simulink model "HyL_SV_test"  (R2013a)
settings: Solver=ode45  StartTime=0.0  StopTime=3  FixedStep=1e-3  MinStep=1e-3  RelTol=1e-3
model workspace (MATLAB code in the model file):
  | % Data obtained from:
  | % ------------------------------------------------------------
  | % HyQ-Robot: Standard Definition for Joint Angles
  | % and Kinematic Parameters of the Legs and Torso
  | %
  | % Project: HyQ-Robot V1.0 with Leg V2.0
  | % Genoa, 9th July 2010
  | %-------------------------------------------------------------
  | % This Matlab file was made by:
  | % Job Ledezma
  | % Genova, Feb 2016
  | %-------------------------------------------------------------
  | 
  | 
  | % ________________________________________
  | %
  | %                HYL DESCRIPTION PARAMETERS
  | %________________________________________
  | 
  | % ---- Leg data ------
  | 
  | m1 = 1.772;              % Kg - Upper leg mass
  | m2 = 0.808;              % Kg - Lower leg mass
  | M = 3.982;                % Kg - Base mass
  | P_01 = 0.08;             % m - distance P0-P1
  | P_12 = 0.350;           % m - distance P1-P2
  | P_23 = 0.330;           % m - distance P2-P3
  | FR = 0.02;                 % m - foot radius
  | P1m1 = 0.164;           % m - distance P1-Pm1
  | P2m2 = 0.122;           % m - distance P2-Pm2
  | I1zz = 0.0713;           % kg·m2 - Inertia upper leg
  | I2zz = 0.0218;           % kg·m2 - Inertia lower leg
  | em1 = deg2rad(7.9);  % rad
  | em2 = deg2rad(0);     % rad
  | g  = 9.810;                 % m/s2 - gravity
  | 
  | % ----- Lever Arm Parameters -----
  | 
  | % Hip joint
  | a1   = 0.3219;             % m
  | b1   = 0.045;               % m
  | e11 = deg2rad(6.24); % rad
  | e12 = deg2rad(0);      % rad
  | 
  | % Knee joint
  | a2 = 0.3218;               % m
  | b2 = 0.045;                 % m
  | e21 = deg2rad(8.04);  % rad
  | e22 = deg2rad(6);       % rad
  | 
  | % ----- Limit Angles --------
  | 
  | % Initial conditions
  | q0_0 = 1;                           % m - height of the floating base
  | q1_0 = deg2rad(45);         % rad - HFE angle
  | q2_0 = deg2rad(-90);        % rad - KFE angle
  | 
  | % Max angle limits
  | q1Max = deg2rad(70);       % rad
  | q2Max = deg2rad(-20);      % rad
  | 
  | % Min angle limits
  | q1Min = deg2rad(-50);        % rad
  | q2Min = deg2rad(-140);      % rad
  | q0Min = P_01+P_12*cos(q1Min)+P_23*cos(q1Min+q2Min)+FR;     % m
  | 
  | % ________________________________________________________
  | %
  | %                                        HYDRAULIC PARAMETERS
  | % ________________________________________________________
  | 
  | % ------ Power unit --------
  | 
  | ps  = 160e5;                            % Pa - Supply pressure
  | pt  = 10e5;                              % Pa - Tank pressure
  | dpt = ps - pt;                           % Pa - Delta pressure
  | beta = 1.4e9;                          % Pa- Effective bulk modulus
  | 
  | % Initial condition for Pressure integrators
  | pAo = ps/2;
  | pBo = ps/2;
  | 
  | %----- Cylinder - HOERBIGER LB6 16 10 0080 4M ----------
  | 
  | Dp = 0.016;                             % m - Piston diameter
  | Dr = 0.010;                              % m - Rod diameter
  | L  = 0.080;                               % m- Stroke
  | Aa = pi*(Dp^2)/4;                   % m^2 - Area A of the piston
  | Ab = pi*(Dp^2-Dr^2)/4;         % m^2 - Area B of the piston
  | r  = Aa/Ab;                              % Relation between areas
  | fv = 700;                                 %  Ns/m - Viscous friction
  | % leak = 1.7*10^-13;            % m3/(s.Pa) - Cylinder leakage
  | Mp = ((pi*Dr^2/4)*L + Aa*0.15)*7860;    % Kg - Piston mass (approximated)
  | 
  | %-----  Valve Parameters - MOOG E024 - 177LA ----------
  | 
  | Un   = 10;                              % V - Nominal tension
  | Qn   = 5 / 60e3;                    % m^3/s - Nominal flow rate
  | dptn = 70e5;                         % Pa - Valve pressure drop
  | Qlk   = 0.28 / 60e3;               % m^3/s - Leakage flow
  | Plk    = 210e5;                       % Pa - Nominal supply pressure for leakage test
  | wn    = 2*32*pi;                    % rad/s - Valve's natural frequency
  | E       = 0.9;                           % Valve's damping coefficient
  | Kv     = Qn/sqrt(dptn);          % m^3/(s*sqrt(Pa)) - Total flow coefficient
  | Kva    = Kv*sqrt(2);               % m^3/(s*sqrt(Pa)) - Partial flow coefficient A
  | Kvb    = Kv*sqrt(2);               % m^3/(s*sqrt(Pa)) - Partial flow coefficient B
  | Kvlk   = Qlk/sqrt(2*Plk);         % m^3/(s*sqrt(Pa)) - Total leakage flow coefficient
  | KvlkA  = Kvlk;                         % m^3/(s*sqrt(Pa)) -  Partial leakage flow coefficient A
  | KvlkB  = Kvlk;                         % m^3/(s*sqrt(Pa)) - Partial leakage flow coefficient B
  | 
  | %------------   Manifold  -----------
  | % Review this part with the manifold's CAD design
  | 
  | v1a = (pi*(0.0035^2)/4)*0.07255;
  | v2a = (pi*(0.006^2)/4)*(0.090-0.012);
  | v1b = (pi*(0.0035^2)/4)*0.04491;
  | v2b = (pi*(0.006^2)/4)*(0.019+0.009);
  | v3b = (pi*(0.006^2)/4)*(0.007+0.009);
  | V0A = v1a + v2a;                                            % Dead volume coupled to chamber A
  | V0B = v1b + v2b + v3b;                                  % Dead volume coupled to chamber B
  | 
  | %-------  Load cell - BURSTER 8417-6005 ----------
  | 
  | xs = 6e-6;                             % m - Maximum deflection @ full scale
  | Fs = 5000;                             % N - Maximum force
  | Ks = Fs / xs ;                         % N·m - Load cell stiffness
  | 
  | %------ Accumulator - FOX-ITALY HST 0,04 ----------
  | 
  | acc = 0;
  | 
  | n = 1.4;                                % Polytropic constant
  | V0 = 0.04e-3;                       % m3 - Initial volume
  | P0 = 120e5 + 1e5;               % Pa - Precharge pressure
  | Cex = 0;                                % m3/Pa - External flowrate coefficient between chambers (in case of damping requirement)
undefined symbols (not defined in the file): Fpt, gcontact, gcPosVel, HyL_Job
libraries: simulink x4
settings Model: Creator=Toshiba  LastModifiedBy=Toshiba
settings SolverCC: ZeroCrossControl=EnableAll  ZeroCrossAlgorithm=Adaptive

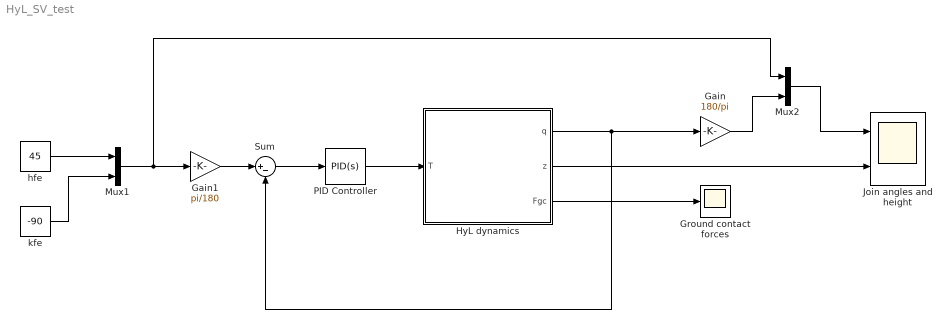
== system HyL_SV_test ==
  Gain : Gain  Gain=180/pi
  Gain1 : Gain  Gain=pi/180
  Ground contact forces : Scope
      settings: SaveName=ScopeData3
  HyL dynamics : Subsystem
  Join angles and height : Scope  NumInputPorts=2
      settings: YMin=-150~-1.14399e-05  YMax=75~-1.03503e-05
  Mux1 : Mux  Inputs=2
  Mux2 : Mux  Inputs=2
  PID Controller : simulink/Continuous/PID Controller  Controller=PID  TimeDomain=Continuous-time  SampleTime=1  IntegratorMethod=Forward Euler  FilterMethod=Forward Euler  Form=Parallel  P=200  I=0  D=6  N=100  InitialConditionSource=internal  InitialConditionForIntegrator=0  InitialConditionForFilter=0  ExternalReset=none  LimitOutput=off  UpperSaturationLimit=inf  LowerSaturationLimit=-inf  LinearizeAsGain=on  AntiWindupMode=none  Kb=1  TrackingMode=off  Kt=1  PParamMin=[]  PParamMax=[]  IParamMin=[]  IParamMax=[]  DParamMin=[]  DParamMax=[]  NParamMin=[]  NParamMax=[]  KbParamMin=[]  KbParamMax=[]  KtParamMin=[]  KtParamMax=[]  POutMin=[]  POutMax=[]  IOutMin=[]  IOutMax=[]  DOutMin=[]  DOutMax=[]  NOutMin=[]  NOutMax=[]  KbOutMin=[]  KbOutMax=[]  KtOutMin=[]  KtOutMax=[]  IntegratorOutMin=[]  IntegratorOutMax=[]  FilterOutMin=[]  FilterOutMax=[]  SumOutMin=[]  SumOutMax=[]  SumI1OutMin=[]  SumI1OutMax=[]  SumI2OutMin=[]  SumI2OutMax=[]  SumI3OutMin=[]  SumI3OutMax=[]  SumDOutMin=[]  SumDOutMax=[]  SaturationOutMin=[]  SaturationOutMax=[]  IntegratorContinuousStateAttributes=''  IntegratorStateMustResolveToSignalObject=off  IntegratorRTWStateStorageClass=Auto  FilterContinuousStateAttributes=''  FilterStateMustResolveToSignalObject=off  FilterRTWStateStorageClass=Auto
  Sum : Sum  Inputs=|+-
  hfe : Constant  Value=45
  kfe : Constant  Value=-90
  wires:
  HyL dynamics/1(q) -> Gain/1, Sum/2
  HyL dynamics/2(z) -> Join angles and height/2
  Mux1/1 -> Mux2/1, Gain1/1
  kfe/1 -> Mux1/2
  hfe/1 -> Mux1/1
  Sum/1 -> PID Controller/1
  Gain1/1 -> Sum/1
  Gain/1 -> Mux2/2
  Mux2/1 -> Join angles and height/1
  HyL dynamics/3(Fgc) -> Ground contact forces/1
  PID Controller/1 -> HyL dynamics/1(T)

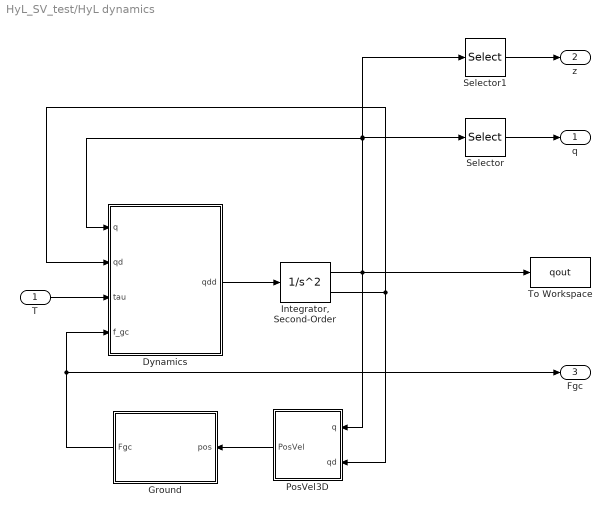
== system HyL_SV_test/HyL dynamics ==
  T : Inport
  Dynamics : Subsystem
  Ground : Subsystem
  "Integrator, Second-Order" : SecondOrderIntegrator  ICX=[q0_0;q1_0;q2_0]  LimitX=on  UpperLimitX=[inf; q1Max; q2Max]  LowerLimitX=[q0Min; q1Min; q2Min]
  PosVel3D : Subsystem
  Selector : Selector  InputPortWidth=3  IndexOptions=Index vector (dialog)  Indices=[2 3]  OutputSizes=1
  Selector1 : Selector  InputPortWidth=3  IndexOptions=Index vector (dialog)  Indices=1  OutputSizes=1
  To Workspace : ToWorkspace  VariableName=qout  SampleTime=-1  SaveFormat=Timeseries
  q : Outport
  z : Outport  Port=2
  Fgc : Outport  Port=3
  wires:
  Dynamics/1(qdd) -> "Integrator, Second-Order"/1
  "Integrator, Second-Order"/1 -> Selector1/1, Selector/1, Dynamics/1(q), To Workspace/1, PosVel3D/1(q)
  "Integrator, Second-Order"/2 -> PosVel3D/2(qd), Dynamics/2(qd)
  Selector/1 -> q/1
  T/1 -> Dynamics/3(tau)
  Selector1/1 -> z/1
  PosVel3D/1(PosVel) -> Ground/1(pos)
  Ground/1(Fgc) -> Fgc/1, Dynamics/4(f_gc)

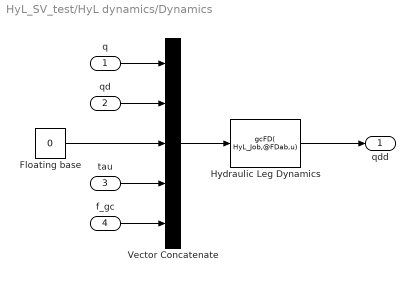
== system HyL_SV_test/HyL dynamics/Dynamics ==
  q : Inport
  qd : Inport  Port=2
  tau : Inport  Port=3
  f_gc : Inport  Port=4
  Floating base : Constant  Value=0
  Hydraulic Leg Dynamics : MATLABFcn  MATLABFcn=gcFD( HyL_Job,@FDab,u)  OutputDimensions=[3 1]  OutputSignalType=real  Output1D=off
  Vector Concatenate : Concatenate  NumInputs=5
  qdd : Outport
  wires:
  Hydraulic Leg Dynamics/1 -> qdd/1
  Vector Concatenate/1 -> Hydraulic Leg Dynamics/1
  qd/1 -> Vector Concatenate/2
  q/1 -> Vector Concatenate/1
  f_gc/1 -> Vector Concatenate/5
  tau/1 -> Vector Concatenate/4
  Floating base/1 -> Vector Concatenate/3

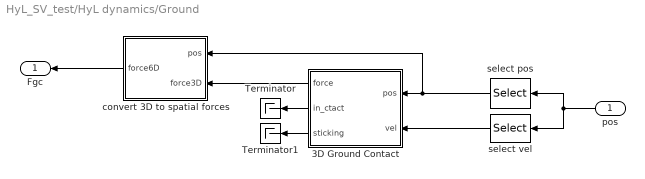
== system HyL_SV_test/HyL dynamics/Ground ==
  pos : Inport
  3D Ground Contact : Subsystem  mask(3D Nonlinear Ground Contact with Friction){K=1e6, D=2000, mu=0.1, np=1}
      mask prompts: K "Stiffness (K)"; D "Damping (D)"; mu "Coefficient of Friction (mu)"; np "Number of Contact Points"
      mask help:
      | Given two 3xnp arrays containing contact-point positions and
      | velocities, calculate the 3xnp array of ground-reaction forces
      | acting on those points. Also calculate 1xnp boolean vectors
      | in_ctact (true if normal force >0) and sticking (true if inside
      | or on boundary of friction cone).  Zero-crossing detection is
      | enabled at both make/break contact and stick/slip transitions.
  Terminator : Terminator
  Terminator1 : Terminator
  convert 3D to spatial forces : Subsystem
  select pos : Selector  NumberOfDimensions=2  InputPortWidth=3  IndexOptions=Index vector (dialog),Select all  Indices=[1 2 3],1  OutputSizes=1,1
  select vel : Selector  NumberOfDimensions=2  InputPortWidth=3  IndexOptions=Index vector (dialog),Select all  Indices=[4 5 6],1  OutputSizes=1,1
  Fgc : Outport
  wires:
  select vel/1 -> 3D Ground Contact/2(vel)
  3D Ground Contact/1(force) -> convert 3D to spatial forces/2(force3D)
  3D Ground Contact/2(in_ctact) -> Terminator/1
  3D Ground Contact/3(sticking) -> Terminator1/1
  convert 3D to spatial forces/1(force6D) -> Fgc/1
  select pos/1 -> convert 3D to spatial forces/1(pos), 3D Ground Contact/1(pos)
  pos/1 -> select vel/1, select pos/1

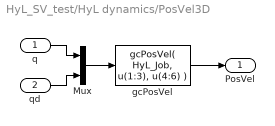
== system HyL_SV_test/HyL dynamics/PosVel3D ==
  q : Inport
  qd : Inport  Port=2
  Mux : Mux  Inputs=2
  gcPosVel : MATLABFcn  MATLABFcn=gcPosVel( HyL_Job, u(1:3), u(4:6) )  OutputDimensions=[6 1]  OutputSignalType=real  Output1D=off
  PosVel : Outport
  wires:
  q/1 -> Mux/1
  qd/1 -> Mux/2
  Mux/1 -> gcPosVel/1
  gcPosVel/1 -> PosVel/1

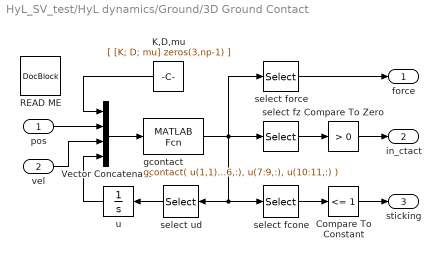
== system HyL_SV_test/HyL dynamics/Ground/3D Ground Contact ==
  pos : Inport
  vel : Inport  Port=2
  Compare To Constant : simulink/Logic and Bit Operations/Compare To Constant  relop=<=  const=1  OutDataTypeStr=boolean
  Compare To Zero : simulink/Logic and Bit Operations/Compare To Zero  relop=>  OutDataTypeStr=boolean
  K,D,mu : Constant  Value=[ [K; D; mu] zeros(3,np-1) ]  VectorParams1D=off
  READ ME : simulink/Model-Wide Utilities/DocBlock  DocumentType=Text
      content=|
      | The constant block supplies the parameters K, D and mu to the function
      | gcontact.  This is necessary because K, D and mu are defined in the
      | workspace of this particular masked subsystem, but the executable
      | expression in the "MATLAB Function" block does not have access to this
      | workspace, so the symbols K, D and mu cannot appear directly in the
      | executable expression.
      |
      | The ">0" block and the "<=1" block both have zero-crossing enabled.  The
      | former detects transitions between contact and non-contact, whereas the
      | latter detects transitions between sticking (due to friction) and
      | slipping.  A point can be sticking only if it is also in contact.  A
      | zero-crossing event occurs whenever any one point makes a transition.
      |
      | The state variable, u, is a 2x(np) matrix containing the horizontal
      | component of the local ground deformation for each point.  This quantity
      | is used to calculate the tangential (i.e., frictional) component of the
      | ground reaction force.
      |
      | When a point loses contact, its associated state variable, u(:,i), decays
      | to zero with a time constant of D/K.  If this ratio is small then the
      | corresponding differential equation is fast, and it is necessary to use
      | small integration time steps.  For example, if K=1e6 and D=2000 then
      | D/K=0.002 and u(:,i) decays in proportion to exp(-500t).  Increasing K
      | makes the surface stiffer, and decreasing D/K makes it bouncier, but the
      | latter also makes the post-contact recovery faster.  The degree of
      | bounciness depends on the mass of the impacting body: a heavier body will
      | bounce more.
      |
      | To adapt this subsystem to work in 2D, the only things that change are the
      | row dimensions of various matrices.  You will have to alter the row
      | selections in the executable expression in the "MATLAB Function" block,
      | and also the dimensions of its output matrix, and you will have to change
      | the row selections in the various "select" blocks.
      |
      | For more information, see "The Simulink Ground Contact Model" in the
      | spatial_v2 documentation directory.
  Vector Concatenate : Concatenate  NumInputs=4  Mode=Multidimensional array
  gcontact : MATLABFcn  MATLABFcn=gcontact( u(1,1), u(2,1), u(3,1), u(4:6,:), u(7:9,:), u(10:11,:) )  OutputDimensions=[6 np]  OutputSignalType=real  Output1D=off
  select fcone : Selector  NumberOfDimensions=2  InputPortWidth=3  IndexOptions=Index vector (dialog),Select all  Indices=[6],1  OutputSizes=1,1
  select force : Selector  NumberOfDimensions=2  InputPortWidth=3  IndexOptions=Index vector (dialog),Select all  Indices=[1 2 3],1  OutputSizes=1,1
  select fz : Selector  NumberOfDimensions=2  InputPortWidth=3  IndexOptions=Index vector (dialog),Select all  Indices=[3],1  OutputSizes=1,1
  select ud : Selector  NumberOfDimensions=2  InputPortWidth=3  IndexOptions=Index vector (dialog),Select all  Indices=[4 5],1  OutputSizes=1,1
  u : Integrator
  force : Outport
  in_ctact : Outport  Port=2
  sticking : Outport  Port=3
  wires:
  Vector Concatenate/1 -> gcontact/1
  select ud/1 -> u/1
  gcontact/1 -> select fz/1, select ud/1, select fcone/1, select force/1
  select force/1 -> force/1
  select fz/1 -> Compare To Zero/1
  Compare To Zero/1 -> in_ctact/1
  select fcone/1 -> Compare To Constant/1
  Compare To Constant/1 -> sticking/1
  u/1 -> Vector Concatenate/4
  vel/1 -> Vector Concatenate/3
  pos/1 -> Vector Concatenate/2
  K,D,mu/1 -> Vector Concatenate/1

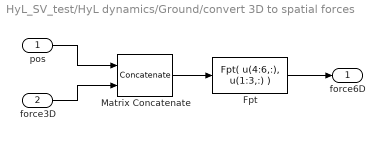
== system HyL_SV_test/HyL dynamics/Ground/convert 3D to spatial forces ==
  pos : Inport
  force3D : Inport  Port=2
  Fpt : MATLABFcn  MATLABFcn=Fpt( u(4:6,:), u(1:3,:) )  OutputSignalType=real  Output1D=off
  Matrix Concatenate : Concatenate  Mode=Multidimensional array
  force6D : Outport
  wires:
  force3D/1 -> Matrix Concatenate/2
  pos/1 -> Matrix Concatenate/1
  Matrix Concatenate/1 -> Fpt/1
  Fpt/1 -> force6D/1
